simulink model "BESS1_pu"  (R2020b)
settings: Solver=ode1  StartTime=0.0  StopTime=160  FixedStep=Ts  RelTol=1e-3
PostLoadFcn:
  | clc; clear all; close all;
  | 
  | % Modulo 10 - Controle Grid-Forming %
  | 
  | vs_ref = 400;
  | Vnom_rms = vs_ref;
  | Vnom_peak = sqrt(2/3)*Vnom_rms;
  | Pnom =29.75e3;
  | Sbase = Pnom;
  | Vdc = 1400;
  | wnom = 2*pi*60;
  | ron = 0.00088;
  | Ron = ron;
  | %%%% To pu %%%%
  | Vbase = Vnom_rms*sqrt(2);
  | V_LG = Vnom_rms/sqrt(3);
  | Ibase = (Pnom*sqrt(2))/(V_LG*3);
  | 
  | Irms = Pnom/(sqrt(3)*Vnom_rms);                     % Ig rms
  | Inom_peak = Irms*sqrt(2);                           % Ig pico
  | Zbase = Vnom_peak/Inom_peak;                        % Impedancia Base
  | Kconv = Zbase;                                      % Ganho conversor
  | 
  | %%%% LCL Filter Project %%%%
  | fsw = 105*60;%105*60;                                         % switching frequency
  | ripple = 0.05;                                       % current ripple
  | L1 = Vdc/(6*ripple*Inom_peak*fsw);                  % inductor L1
  | R1 = 0.005;                                        % L1 resistance
  | Cbase = 1/(wnom*Kconv);                             % base capacitance
  | Cf = 0.05*Cbase;                                    % filter capacitor
  | Cf = 400e-6;
  | 
  | 
  | % Capacitor DC
  | C_cc_proj = (Sbase/(2*pi*60*Vdc*Vdc*0.05));
  | 
  | % Controladores
  | tau_i = 0.0005;
  | kp_corrente = L1/tau_i
  | ki_corrente = (R1+ron)/tau_i
  | kp_current_pu = kp_corrente/Kconv;                  % Adaptando para pu
  | ki_current_pu = ki_corrente/Kconv;
  | decouple_pu = (wnom*L1+(R1+Ron))/Kconv;
  | 
  | %decouple_i = wnom*L1
  | decouple_v = wnom*Cf
  | decouple_v_pu = (wnom*Cf)*Kconv;
  | 
  | % Controlador CA
  | S_Load = sqrt((25e3)^2+(20e3)^2);
  | Ibase_Load = ((S_Load*sqrt(2))/(V_LG*3))
  | 
  | 
  | a1=2
  | kp_tensao = Cf/(a1*tau_i)
  | Tn = 4*tau_i;
  | ki_tensao = kp_tensao/Tn
  | 
  | % To pu
  | Ica_pu = Pnom/Vdc;
  | %Kcc = Vdc/Iext;
  | 
  | 
  | 
  | 
  | a2=(1+(2/sqrt(2)))
  | kp_tensao2 = Cf/(a2*tau_i)
  | ki_tensao2 = kp_tensao2/Tn
  | 
  | 
  | Ts =25e-6; Ts_Control=Ts;
  | 
  | % PR_ideal_tensao = tf([2*ki_tensao],[1 0 (w^2)]);
  | % PR_ideal_corrente = tf([2*ki_corrente],[1 0 (w^2)]);
  | % figure(1)
  | % bode(PR_ideal_tensao)
  | %
  | % wc = 5;
  | %
  | % PR_real = tf([2*ki_tensao*wc],[1 2*wc (w^2)]);
  | % figure(2)
  | % bode(PR_real)
  | %
  | % wc1 = 1;
  | %
  | % PR_real1 = tf([2*ki_tensao*wc1],[1 2*wc1 (w^2)]);
  | % figure(3)
  | % bode(PR_real1)
InitFcn:
  | clc; clear all; close all;
  | 
  | % Modulo 10 - Controle Grid-Forming %
  | 
  | vs_ref = 400;
  | Vnom_rms = vs_ref;
  | Vnom_peak = sqrt(2/3)*Vnom_rms;
  | Pnom =29.75e3;
  | Sbase = Pnom;
  | Vdc = 1400;
  | wnom = 2*pi*60;
  | ron = 0.00088;
  | Ron = ron;
  | %%%% To pu %%%%
  | Vbase = Vnom_rms*sqrt(2);
  | V_LG = Vnom_rms/sqrt(3);
  | Ibase = (Pnom*sqrt(2))/(V_LG*3);
  | 
  | Irms = Pnom/(sqrt(3)*Vnom_rms);                     % Ig rms
  | Inom_peak = Irms*sqrt(2);                           % Ig pico
  | Zbase = Vnom_peak/Inom_peak;                        % Impedancia Base
  | Kconv = Zbase;                                      % Ganho conversor
  | 
  | %%%% LCL Filter Project %%%%
  | fsw = 105*60;%105*60;                                         % switching frequency
  | ripple = 0.05;                                       % current ripple
  | L1 = Vdc/(6*ripple*Inom_peak*fsw);                  % inductor L1
  | R1 = 0.005;                                        % L1 resistance
  | Cbase = 1/(wnom*Kconv);                             % base capacitance
  | Cf = 0.05*Cbase;                                    % filter capacitor
  | Cf = 400e-6;
  | 
  | 
  | % Capacitor DC
  | C_cc_proj = (Sbase/(2*pi*60*Vdc*Vdc*0.05));
  | 
  | % Controladores
  | tau_i = 0.0005;
  | kp_corrente = L1/tau_i
  | ki_corrente = (R1+ron)/tau_i
  | kp_current_pu = kp_corrente/Kconv;                  % Adaptando para pu
  | ki_current_pu = ki_corrente/Kconv;
  | decouple_pu = (wnom*L1+(R1+Ron))/Kconv;
  | 
  | %decouple_i = wnom*L1
  | decouple_v = wnom*Cf
  | decouple_v_pu = (wnom*Cf)*Kconv;
  | 
  | % Controlador CA
  | S_Load = sqrt((25e3)^2+(20e3)^2);
  | Ibase_Load = ((S_Load*sqrt(2))/(V_LG*3))
  | 
  | 
  | a1=2
  | kp_tensao = Cf/(a1*tau_i)
  | Tn = 4*tau_i;
  | ki_tensao = kp_tensao/Tn
  | 
  | % To pu
  | Ica_pu = Pnom/Vdc;
  | %Kcc = Vdc/Iext;
  | 
  | 
  | 
  | 
  | a2=(1+(2/sqrt(2)))
  | kp_tensao2 = Cf/(a2*tau_i)
  | ki_tensao2 = kp_tensao2/Tn
  | 
  | 
  | Ts =25e-6; Ts_Control=Ts;
  | 
  | % PR_ideal_tensao = tf([2*ki_tensao],[1 0 (w^2)]);
  | % PR_ideal_corrente = tf([2*ki_corrente],[1 0 (w^2)]);
  | % figure(1)
  | % bode(PR_ideal_tensao)
  | %
  | % wc = 5;
  | %
  | % PR_real = tf([2*ki_tensao*wc],[1 2*wc (w^2)]);
  | % figure(2)
  | % bode(PR_real)
  | %
  | % wc1 = 1;
  | %
  | % PR_real1 = tf([2*ki_tensao*wc1],[1 2*wc1 (w^2)]);
  | % figure(3)
  | % bode(PR_real1)
StartFcn:
  | clc; clear all; close all;
  | 
  | % Modulo 10 - Controle Grid-Forming %
  | 
  | vs_ref = 400;
  | Vnom_rms = vs_ref;
  | Vnom_peak = sqrt(2/3)*Vnom_rms;
  | Pnom =29.75e3;
  | Sbase = Pnom;
  | Vdc = 1400;
  | wnom = 2*pi*60;
  | ron = 0.00088;
  | Ron = ron;
  | %%%% To pu %%%%
  | Vbase = Vnom_rms*sqrt(2);
  | V_LG = Vnom_rms/sqrt(3);
  | Ibase = (Pnom*sqrt(2))/(V_LG*3);
  | 
  | Irms = Pnom/(sqrt(3)*Vnom_rms);                     % Ig rms
  | Inom_peak = Irms*sqrt(2);                           % Ig pico
  | Zbase = Vnom_peak/Inom_peak;                        % Impedancia Base
  | Kconv = Zbase;                                      % Ganho conversor
  | 
  | %%%% LCL Filter Project %%%%
  | fsw = 105*60;%105*60;                                         % switching frequency
  | ripple = 0.05;                                       % current ripple
  | L1 = Vdc/(6*ripple*Inom_peak*fsw);                  % inductor L1
  | R1 = 0.005;                                        % L1 resistance
  | Cbase = 1/(wnom*Kconv);                             % base capacitance
  | Cf = 0.05*Cbase;                                    % filter capacitor
  | Cf = 400e-6;
  | 
  | 
  | % Capacitor DC
  | C_cc_proj = (Sbase/(2*pi*60*Vdc*Vdc*0.05));
  | 
  | % Controladores
  | tau_i = 0.0005;
  | kp_corrente = L1/tau_i
  | ki_corrente = (R1+ron)/tau_i
  | kp_current_pu = kp_corrente/Kconv;                  % Adaptando para pu
  | ki_current_pu = ki_corrente/Kconv;
  | decouple_pu = (wnom*L1+(R1+Ron))/Kconv;
  | 
  | %decouple_i = wnom*L1
  | decouple_v = wnom*Cf
  | decouple_v_pu = (wnom*Cf)*Kconv;
  | 
  | % Controlador CA
  | S_Load = sqrt((25e3)^2+(20e3)^2);
  | Ibase_Load = ((S_Load*sqrt(2))/(V_LG*3))
  | 
  | 
  | a1=2
  | kp_tensao = Cf/(a1*tau_i)
  | Tn = 4*tau_i;
  | ki_tensao = kp_tensao/Tn
  | 
  | % To pu
  | Ica_pu = Pnom/Vdc;
  | %Kcc = Vdc/Iext;
  | 
  | 
  | 
  | 
  | a2=(1+(2/sqrt(2)))
  | kp_tensao2 = Cf/(a2*tau_i)
  | ki_tensao2 = kp_tensao2/Tn
  | 
  | 
  | Ts =25e-6; Ts_Control=Ts;
  | 
  | % PR_ideal_tensao = tf([2*ki_tensao],[1 0 (w^2)]);
  | % PR_ideal_corrente = tf([2*ki_corrente],[1 0 (w^2)]);
  | % figure(1)
  | % bode(PR_ideal_tensao)
  | %
  | % wc = 5;
  | %
  | % PR_real = tf([2*ki_tensao*wc],[1 2*wc (w^2)]);
  | % figure(2)
  | % bode(PR_real)
  | %
  | % wc1 = 1;
  | %
  | % PR_real1 = tf([2*ki_tensao*wc1],[1 2*wc1 (w^2)]);
  | % figure(3)
  | % bode(PR_real1)
undefined symbols (not defined in the file): DiscIntNeverNeededParam, I, Ion, Left, Lithium, ph, type, V
libraries: powerlib x18, powerlib_meascontrol x16, rtlab x6, artemis x2, eePowerMeasurement x2, rteventslib x2, ssn_inverter_model x1, electricdrivelib x1
(part 1 of 2)
settings Model: ARTEMISmethode_block_infos=$$__separator__$$BESS1_pu/ARTEMIS Guide$$__separator__$$  Creator=Lafae  LastModifiedBy=lafae
settings DataIOCC: SaveOutput=off  SaveTime=off  ReturnWorkspaceOutputs=off
settings OptimizationCC: BlockReduction=off  OptimizeBlockIOStorage=off  BufferReuse=off  GlobalBufferReuse=off  ExpressionFolding=off  LocalBlockOutputs=off  OptimizeDataStoreBuffers=off  BusAssignmentInplaceUpdate=off
settings DebuggingCC: ArithmeticOperatorsInVariantConditions=warning
settings SFSimCC: CustomCodeUndefinedFunction=UseInterfaceOnly

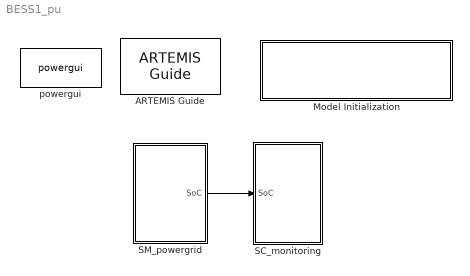
== system BESS1_pu ==
  ARTEMIS Guide : artemis/ARTEMIS/ARTEMIS Guide  Tag=art7.5  Description=New ARTEMiS block v 7.5b (R2015b+)  lock=on  Ts=Ts  ssn=on  opt=art5  dyna=off  nb_perm=4  RT_fullcomp=off  ssn_itvc=off  ssn_ivic=off  ssn_ext=off  ssn_solver=Art5  iter_type=iSWITCH and iMOV only (default)  ssn_ImpulseLoopBlockedStateUpdate=5  ssn_mov_iter_number=5  ssn_switch_iter_number=3  ssn_lu_or_ldlt=LU (more robust)  ssn_nib_type_verify=on  ssn_use_lu=on  ssn_use_ldlt=off  ssn_impulse=on  ssn_quasimpulse=off  ssn_impulse_loop=5  paraExtinctionThy=off  Thy_Impulse=on  dtc=Off  dtc_opt=normal  ao=off  simtype=off  ct_mac=off  lin_mov=off  lsp=[0.001 2]  spike_skip=Disabled  dtc_extra=1  dtc_sws=normal  dtc_pied=0.5  SPSRulesBlock=SPSRules  tre=off  ctmm=off  LF=off  dpl_type=ARTEMiS DPL  rlc_type=off  custom_type=off  para=on  ssn_full_iteration=off  ssn_init_cond=block only
  Model Initialization : Subsystem  AncestorBlock=artemis/Tools /Misc/Model Initialization  mask(Model Functions){InitFcnX=|, prel=off, posl=on, inif=on, strf=on}
      mask InitFcnX=|
      | clc; clear all; close all;
      |
      | % Modulo 10 - Controle Grid-Forming %
      |
      | vs_ref = 400;
      | Vnom_rms = vs_ref;
      | Vnom_peak = sqrt(2/3)*Vnom_rms;
      | Pnom =29.75e3;
      | Sbase = Pnom;
      | Vdc = 1400;
      | wnom = 2*pi*60;
      | ron = 0.00088;
      | Ron = ron;
      | %%%% To pu %%%%
      | Vbase = Vnom_rms*sqrt(2);
      | V_LG = Vnom_rms/sqrt(3);
      | Ibase = (Pnom*sqrt(2))/(V_LG*3);
      |
      | Irms = Pnom/(sqrt(3)*Vnom_rms);                     % Ig rms
      | Inom_peak = Irms*sqrt(2);                           % Ig pico
      | Zbase = Vnom_peak/Inom_peak;                        % Impedancia Base
      | Kconv = Zbase;                                      % Ganho conversor
      |
      | %%%% LCL Filter Project %%%%
      | fsw = 105*60;%105*60;                                         % switching frequency
      | ripple = 0.05;                                       % current ripple
      | L1 = Vdc/(6*ripple*Inom_peak*fsw);                  % inductor L1
      | R1 = 0.005;                                        % L1 resistance
      | Cbase = 1/(wnom*Kconv);                             % base capacitance
      | Cf = 0.05*Cbase;                                    % filter capacitor
      | Cf = 400e-6;
      |
      |
      | % Capacitor DC
      | C_cc_proj = (Sbase/(2*pi*60*Vdc*Vdc*0.05));
      |
      | % Controladores
      | tau_i = 0.0005;
      | kp_corrente = L1/tau_i
      | ki_corrente = (R1+ron)/tau_i
      | kp_current_pu = kp_corrente/Kconv;                  % Adaptando para pu
      | ki_current_pu = ki_corrente/Kconv;
      | decouple_pu = (wnom*L1+(R1+Ron))/Kconv;
      |
      | %decouple_i = wnom*L1
      | decouple_v = wnom*Cf
      | decouple_v_pu = (wnom*Cf)*Kconv;
      |
      | % Controlador CA
      | S_Load = sqrt((25e3)^2+(20e3)^2);
      | Ibase_Load = ((S_Load*sqrt(2))/(V_LG*3))
      |
      |
      | a1=2
      | kp_tensao = Cf/(a1*tau_i)
      | Tn = 4*tau_i;
      | ki_tensao = kp_tensao/Tn
      |
      | % To pu
      | Ica_pu = Pnom/Vdc;
      | %Kcc = Vdc/Iext;
      |
      |
      |
      |
      | a2=(1+(2/sqrt(2)))
      | kp_tensao2 = Cf/(a2*tau_i)
      | ki_tensao2 = kp_tensao2/Tn
      |
      |
      | Ts =25e-6; Ts_Control=Ts;
      |
      | % PR_ideal_tensao = tf([2*ki_tensao],[1 0 (w^2)]);
      | % PR_ideal_corrente = tf([2*ki_corrente],[1 0 (w^2)]);
      | % figure(1)
      | % bode(PR_ideal_tensao)
      | %
      | % wc = 5;
      | %
      | % PR_real = tf([2*ki_tensao*wc],[1 2*wc (w^2)]);
      | % figure(2)
      | % bode(PR_real)
      | %
      | % wc1 = 1;
      | %
      | % PR_real1 = tf([2*ki_tensao*wc1],[1 2*wc1 (w^2)]);
      | % figure(3)
      | % bode(PR_real1)
      mask prompts: InitFcnX "Initialisation"; prel "Preload Function"; posl "PostLoad Function"; inif "InitFcn"; strf "StartFcn"
      mask init:
      | currentBlock = gcb;
      | root = bdroot(currentBlock);
      | 
      | if ~strcmp(get_param(root,'BlockDiagramType'),'library')
      |     if prel==1
      |         set_param(root, 'PreLoadFcn', InitFcnX);
      |     else
      |         set_param(root, 'PreLoadFcn', '');
      |     end
      |     if inif==1
      |         set_param(root, 'InitFcn', InitFcnX);
      |     else
      |         set_param(root, 'InitFcn', '');
      |     end
      |     if strf==1
      |         set_param(root, 'StartFcn', InitFcnX);
      |     else
      |         set_param(root, 'StartFcn', '');
      |     end
      |     if posl==1
      |         set_param(root, 'PostLoadFcn', InitFcnX);
      |     else
      |         set_param(root, 'PostLoadFcn', '');
      |     end
      | end
      | 
      | pos = get_param(currentBlock, 'Position');
      | width = pos(3) - pos(1); height = pos(4) - pos(2);
      | txt = [ upper(root) '\n' '- InitFcn. . . . . '  get_param(root, 'InitFcn') ];
      settings: CopyFcn=set_param(gcb,'LinkStatus','inactive')
      mask Display: text(5, height*0.5, txt, 'horizontalAlignment', 'left', 'verticalAlignment', 'middle') ;
  SC_monitoring : Subsystem
  SM_powergrid : Subsystem
  powergui : powerlib/powergui  Priority=1  SimulationMode=Discrete  SampleTime=Ts  frequency=60  Iterations=50  frequencyindice=0  Pbase=100e6  ErrMax=1e-4  UnitsV=kV  UnitsW=MW  buscounter=0  FunctionMessages=off  echomessages=off  EnableUseOfTLC=off  CurrentSourceSwitches=off  DisableSnubberDevices=off  DisableRonSwitches=off  DisableVfSwitches=off  DisplayEquations=off  AutomaticDiscreteSolvers=off  SolverType=Tustin/Backward Euler (TBE)  Interpol=off  ExternalGateDelay=off  methode=off  Ts=100  x0status=blocks  SPID=off  SwTol=0  HookPort=off  NonlinearTolerance=1e-4  nMaxIteration=100  ContinueOnMaxIteration=off  RestoreLinks=warning  ResistiveCurrentMeasurement=off  Frange=[0:2:500]  Ylog=off  Xlog=on  ShowGrid=off  save=off  variable=ZData  structure=0  ZoomFFT=off  StartTime=0.0  cycles=1  DisplayStyle=1  fundamental=60  FreqAxis=off  MaxFrequency=1000  frequencyindicesteady=1  RmsSteady=1  display=off
  wires:
  SM_powergrid/1(SoC) -> SC_monitoring/1(SoC)

== system BESS1_pu/Model Initialization ==

== system BESS1_pu/SC_monitoring ==
  SoC : Inport
  OpComm : rtlab/OpComm  nbport=1  groupe_acq=1  subsys_rate=0  st=0  Synchronization=on  Interpolation=on  Threshold=1.0  Missed_Data=off  Sim_Time=off  Samples=off  dynSigOut=off  from_console=0  warning_done=off  writeOpCommFile=off  Offset=off
      settings: SourceProductName=RT-LAB
  SoC_m : Scope
  wires:
  SoC/1 -> OpComm/1
  OpComm/1 -> SoC_m/1

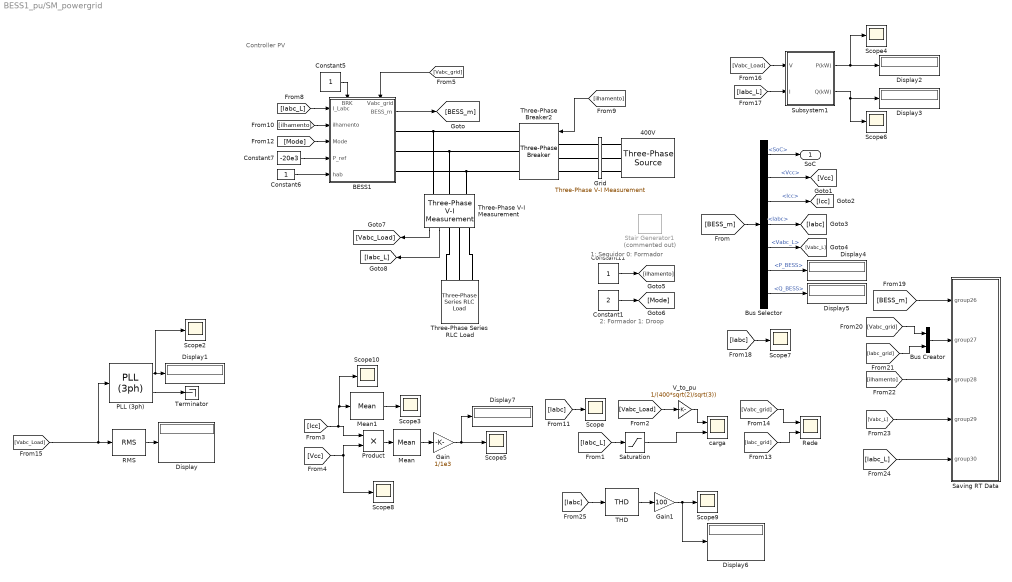
== system BESS1_pu/SM_powergrid ==
  note: Controller PV
  note: 1: Seguidor
      | 0: Formador
  note: 2: Formador
      | 1: Droop
  "400V " : powerlib/Electrical Sources/Three-Phase Source  InternalConnection=Yg  VoltagePhases=off  Voltage=400  PhaseAngle=0  Voltage_phases=[25e3 25e3 25e3]/sqrt(3)  PhaseAngles_phases=[0 -120 +120]  Frequency=60  NonIdealSource=on  SpecifyImpedance=on  Resistance=0.8929  Inductance=16.58e-3  ShortCircuitLevel=2500e6  BaseVoltage=400  XRratio=7  BusType=swing  Pref=0  Qref=0  Prefabc=[10e3, 10e3, 10e3]  Qrefabc=[0, 0, 0]  Qmin=-inf  Qmax=inf
  BESS1 : Subsystem  mask{Parameter1=0, Vdc=1400}
      mask prompts: Parameter1 "Active Power"; Vdc "Voltage BESS"
      settings: PortSchema="{\"entries\":[{\"content\":{\"sides\":[{\"content\":{\"connectorIds\":[\"In1\",\"In2\",\"In3\",\"In4\",\"In5\"]},\"type\":\"ConnectorPlacement.EquallySpacedRectSide\",\"uuid\":\"b852895c-1a88-46a2-b5c3-3793c2bbfa50\"},{\"content\":{\"connectorIds\":[\"Out1\",\"RConn1\",\"RConn2\",\"RConn3\"],\"side\":\"RIGHT\"},\"type\":\"ConnectorPlacement.EquallySpacedRectSide\",\"uuid\":\"623e2f3e-e54c-4c45-bbde-85363be8e45a\"},{\"content\":{\"connectorIds\":[\"In6\",\"In7\"],\"side\":\"TOP\"},\"type\":\"ConnectorPlacement.EquallySpacedRectSide\",\"uuid\":\"4361bef1-4271-4d53-bf17-8738c4288524\"},{\"content\":{\"connectorIds\":[],\"side\":\"BOTTOM\"},\"type\":\"ConnectorPlacement.EquallySpacedRectSide\",\"uuid\":\"fccd725a-212e-4f4d-86e2-af3e4cb1e181\"},{\"content\":{\"connectorIds\":[],\"side\":\"HIDDEN\"},\"type\":\"ConnectorPlacement.EquallySpacedRectSide\",\"uuid\":\"18fd8fa2-4388-4fef-bc52-b43f49f76590\"}]},\"type\":\"ConnectorPlacement.EquallySpacedConnector\",\"uuid\":\"f9b6b572-f2f1-4797-9202-fef1628d084a\"}],\"packageUris\":[\"http://schema.mathworks.com/mf0/Connector/R2020b\"],\"version\":\"1.0\"}"
      mask Display:
      | %image('$imagefile'); % Use "Edit Image" on toolstrip to change.
      | 
      | port_label('input',1,'I_Labc')
      | port_label('input',2,'ilha')
      | port_label('input',3,'Mode')
      | port_label('input',4,'P_ref')
      | port_label('input',5,'hab')
      | port_label('input',6,'BRK')
      | 
      | %output
      | port_label('output',1,'PBESS_m')
      | 
      | %electrical
      | port_label('Rconn',1,'Va')
      | port_label('Rconn',2,'Vb')
      | port_label('Rconn',3,'Vc')
  Bus Creator : BusCreator  Inputs=2
  Bus Selector : BusSelector  OutputSignals=SoC,Vcc,Icc,Iabc,Vabc_L,P_BESS,Q_BESS
  Constant1 : Constant  Value=2
  Constant11 : Constant
  Constant5 : Constant
  Constant6 : Constant
  Constant7 : Constant  Value=-20e3
  Display{,1..7} (8 alike) : Display
  Gain : Gain  Gain=1/1e3
  Gain1 : Gain  Gain=100
  Grid : powerlib/Measurements/Three-Phase V-I Measurement  VoltageMeasurement=phase-to-ground  SetLabelV=on  LabelV=Vabc_grid  Vpu=off  VpuLL=off  CurrentMeasurement=yes  SetLabelI=on  LabelI=Iabc_grid  Ipu=off  Pbase=100e6  Vbase=500e3  OutputType=Complex  PhasorSimulation=off  PSBequivalent=0
  Mean : powerlib_meascontrol/Measurements/Mean  Freq=60  Vinit=0  Ts=0
  Mean1 : powerlib_meascontrol/Measurements/Mean  Freq=60  Vinit=0  Ts=0
  PLL (3ph) : powerlib_meascontrol/PLL/PLL (3ph)  Fmin=45  Par_Init="[-0.57  60]"  ParK=[180, 3200, 1]  TcD=Ts  MaxRateChangeFreq=12  FilterCutOffFreq=25  Ts=Ts  AGC=on
  Product : Product
  RMS : powerlib_meascontrol/Measurements/RMS  TrueRMS=on  Freq=60  RMSInit=1  Ts=Ts
  Rede : Scope  NumInputPorts=2
  Saturation : Saturate  UpperLimit=100  LowerLimit=-100
  Saving RT Data : Subsystem  mask{Ts=Ts, Decimation26=3, varname26=BESS_m, Filename26=BESS.mat, nls26=38, ld26=40, Decimation27=3, varname27=Grid_m, Filename27=Grid.mat, nls27=15, ld27=40, Decimation28=3, varname28=cmd_isla, Filename28=cmd_BRK.mat, nls28=19, ld28=40, Decimation29=3, varname29=Vabc_L, Filename29=Vabc_L.mat, nls29=19, ld29=40, Decimation30=3, varname30=Iabc_L, Filename30=Iabc_L.mat, nls30=20, ld30=40}
      mask prompts: Ts "Ts (s)"; Decimation26 "Decimation factor"; varname26 "Variable name"; Filename26 "FileName"; nls26 "Number of logged signals"; ld26 "Logging duration (s)"; Decimation27 "Decimation factor"; varname27 "Variable name"; Filename27 "FileName"; nls27 "Number of logged signals"; ld27 "Logging duration (s)"; Decimation28 "Decimation factor"; varname28 "Variable name"; Filename28 "FileName"; nls28 "Number of logged signals"; ld28 "Logging duration (s)"; Decimation29 "Decimation factor"; varname29 "Variable name"; Filename29 "FileName"; nls29 "Number of logged signals"; ld29 "Logging duration (s)"; Decimation30 "Decimation factor"; varname30 "Variable name"; Filename30 "FileName"; nls30 "Number of logged signals"; ld30 "Logging duration (s)"
      mask help: This block contains the 5 groups of OpWriteFile (26, 27, 28 29 and 30) blocks that write signals to a binary file (.mat), files that are in the binary data container format that MATLAB uses.
      mask TypeOptions Decimation26: OpWriteFile26/Decimation
      mask TypeOptions varname26: OpWriteFile26/varname
      mask TypeOptions Filename26: OpWriteFile26/Filename
      mask TypeOptions Decimation27: OpWriteFile27/Decimation
      mask TypeOptions varname27: OpWriteFile27/varname
      mask TypeOptions Filename27: OpWriteFile27/Filename
      mask TypeOptions Decimation28: OpWriteFile28/Decimation
      mask TypeOptions varname28: OpWriteFile28/varname
      mask TypeOptions Filename28: OpWriteFile28/Filename
      mask TypeOptions Decimation29: OpWriteFile29/Decimation
      mask TypeOptions varname29: OpWriteFile29/varname
      mask TypeOptions Filename29: OpWriteFile29/Filename
      mask TypeOptions Decimation30: OpWriteFile30/Decimation
      mask TypeOptions varname30: OpWriteFile30/varname
      mask TypeOptions Filename30: OpWriteFile30/Filename
      mask DialogControl DescGroupVar Prompt: Saving RT Data
      mask DialogControl Container4 Prompt: Group 26
      mask DialogControl Container9 Prompt: Group 27
      mask DialogControl Container10 Prompt: Group 28
      mask DialogControl Container11 Prompt: Group 29
      mask DialogControl Container12 Prompt: Group 30
  Scope{,2..10} (10 alike) : Scope
  Stair Generator1 : powerlib_meascontrol/Pulse & Signal Generators/Stair Generator  Commented=on  t=[0, 5, 30, 66]  e=[0, 1, 0, 1]  Ts=0
  Subsystem1 : Subsystem
  THD : powerlib_meascontrol/Measurements/THD  Freq=60  Ts=0
  Terminator : Terminator
  Three-Phase Series RLC Load : powerlib/Elements/Three-Phase Series RLC Load  LConnTagsString=A|B|C  Configuration=Y (grounded)  NominalVoltage=400  Vabc=[1e3 1e3 1e3]  Vabcp=[1e3 1e3 1e3]  NominalFrequency=60  UnbalancedPower=off  ActivePower=25e3  InductivePower=20e3  CapacitivePower=0  Pabc=[10e3 9e3 11e3]  QLabc=[100 90 110]  QCabc=[100 90 110]  Pabcp=[10e3 9e3 11e3]  QLabcp=[100 90 110]  QCabcp=[100 90 110]  Measurements=None  LoadType=constant Z
  Three-Phase V-I Measurement : powerlib/Measurements/Three-Phase V-I Measurement  VoltageMeasurement=phase-to-ground  SetLabelV=off  LabelV=Vabc  Vpu=off  VpuLL=off  CurrentMeasurement=yes  SetLabelI=off  LabelI=Iabc  Ipu=off  Pbase=100e6  Vbase=500e3  OutputType=Complex  PhasorSimulation=off  PSBequivalent=0
  Three-Phase Breaker2 : powerlib/Elements/Three-Phase Breaker  InitialState=open  SwitchA=on  SwitchB=on  SwitchC=on  SwitchTimes=[10]  External=on  BreakerResistance=0.001  SnubberResistance=1e6  SnubberCapacitance=inf  Measurements=None
  V_to_pu : Gain  Gain=1/(400*sqrt(2)/sqrt(3))  SaturateOnIntegerOverflow=on  OutDataTypeStr=Inherit: Same as input  ParamDataTypeStr=Inherit: Same as input
  carga : Scope  NumInputPorts=2
  SoC : Outport
  wires:
  [Icc] -> Scope10/1, Mean1/1, Product/1
  [Vcc] -> Scope8/1, Product/2
  Product/1 -> Mean/1
  Mean/1 -> Gain/1
  Gain/1 -> Display7/1, Scope5/1
  [ilhamento] -> Three-Phase Breaker2/1
  [Iabc] -> Scope/1
  [Iabc_grid] -> Rede/2
  [Vabc_grid] -> Rede/1
  Constant11/1 -> [ilhamento]
  BESS1/1(BESS_m) -> [BESS_m]
  [BESS_m] -> Bus Selector/1
  Bus Selector/1 -> SoC/1  "<SoC>"
  Bus Selector/2 -> [Vcc]  "<Vcc>"
  Bus Selector/3 -> [Icc]  "<Icc>"
  Bus Selector/4 -> [Iabc]  "<Iabc>"
  Bus Selector/5 -> [Vabc_L]  "<Vabc_L>"
  Constant1/1 -> [Mode]
  Constant5/1 -> BESS1/6(BRK)
  [Iabc_L] -> BESS1/1(I_Labc)
  [ilhamento] -> BESS1/2(ilhamento)
  [Mode] -> BESS1/3(Mode)
  Constant7/1 -> BESS1/4(P_ref)
  Constant6/1 -> BESS1/5(hab)
  [Vabc_Load] -> PLL (3ph)/1, RMS/1
  RMS/1 -> Display/1
  PLL (3ph)/2 -> Terminator/1
  PLL (3ph)/1 -> Scope2/1, Display1/1
  Three-Phase V-I Measurement/1 -> [Vabc_Load]
  Three-Phase V-I Measurement/2 -> [Iabc_L]
  [Iabc_L] -> Saturation/1
  Saturation/1 -> carga/2
  [Vabc_Load] -> Subsystem1/1(V)
  [Iabc_L] -> Subsystem1/2(I)
  Subsystem1/1(P(kW)) -> Scope4/1, Display2/1
  Subsystem1/2(Q(kW)) -> Display3/1, Scope6/1
  [Iabc] -> Scope7/1
  Bus Selector/6 -> Display4/1  "<P_BESS>"
  Bus Selector/7 -> Display5/1  "<Q_BESS>"
  Mean1/1 -> Scope3/1
  [BESS_m] -> Saving RT Data/1(group26)
  [Iabc_grid] -> Bus Creator/2
  [Vabc_grid] -> Bus Creator/1
  Bus Creator/1 -> Saving RT Data/2(group27)
  [ilhamento] -> Saving RT Data/3(group28)
  [Vabc_L] -> Saving RT Data/4(group29)
  [Iabc_L] -> Saving RT Data/5(group30)
  [Iabc] -> THD/1
  THD/1 -> Gain1/1
  Gain1/1 -> Display6/1, Scope9/1
  [Vabc_grid] -> BESS1/7(Vabc_grid)
  [Vabc_Load] -> V_to_pu/1
  V_to_pu/1 -> carga/1
  connections:
  Three-Phase V-I Measurement/LConn2 -- Three-Phase Breaker2/RConn2 -- BESS1/RConn2
  Three-Phase V-I Measurement/LConn1 -- BESS1/RConn1 -- Three-Phase Breaker2/RConn1
  Grid/LConn2 -- Three-Phase Breaker2/LConn2
  Grid/LConn1 -- Three-Phase Breaker2/LConn1
  Three-Phase Breaker2/LConn3 -- Grid/LConn3
  "400V "/RConn2 -- Grid/RConn2
  "400V "/RConn3 -- Grid/RConn3
  "400V "/RConn1 -- Grid/RConn1
  Three-Phase V-I Measurement/LConn3 -- BESS1/RConn3 -- Three-Phase Breaker2/RConn3
  Three-Phase Series RLC Load/LConn1 -- Three-Phase V-I Measurement/RConn1
  Three-Phase Series RLC Load/LConn2 -- Three-Phase V-I Measurement/RConn2
  Three-Phase Series RLC Load/LConn3 -- Three-Phase V-I Measurement/RConn3

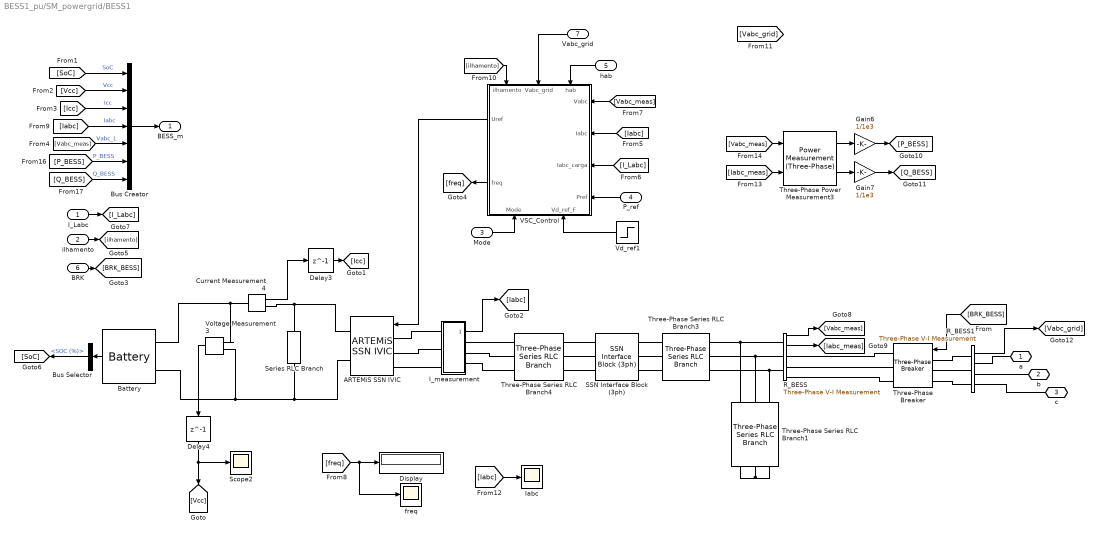
== system BESS1_pu/SM_powergrid/BESS1 ==
  I_Labc : Inport
  ilhamento : Inport  Port=2
  Mode : Inport  Port=3
  P_ref : Inport  Port=4
  hab : Inport  Port=5
  BRK : Inport  Port=6
  Vabc_grid : Inport  Port=7
  ARTEMiS SSN IVIC : ssn_inverter_model/ARTEMiS SSN IVIC  Arms=3  SnubberResistance=800  SnubberCapacitance=inf  Device=IGBT / Diodes  Ron=0.00088  Lon=0  ForwardVoltages=[0.001 0.001]  ForwardVoltage=0  GTOparameters=[ 10e-6 , 20e-6 ]  IGBTparameters=[ 1e-6 , 2e-6 ]*0  Measurements=None  Measurements_2=None  converterType=Rectifier
  Battery : electricdrivelib/Extra Sources/Battery  BatType=Lithium-Ion  ShowTempParam=off  ThermalPreset=no  ShowAgeParam=off  NomV=1400  NomQ=2  SOC=50  Batt_Tr=30  PresetModel=on  MaxQ=2  MinV=1050  FullV=1629.582  Dis_rate=0.86957  R=7  Normal_OP=1.8087  expZone="[1512.5402     0.09826087]"  current=[8 23 32.5]  Units=Time  Tci=20  NomT=20  T2=-30  MaxQ2=4.8  FullV2=7.1  Normal_OP2=5.655  expZone2="[6.58           1]"  Rca=0.6  ti=2000  Dp=0  Neq0=0  Tsim=1e6  Ta1=25  Qeol=5.4*0.9  Reol=0.013333*1.2  Char_age=[2.3478, 3]  Dis_age=[2.3478, 10]  N1=1500  N2=10500  N3=1000  N4=1400  Ta2=45  N5=950
  Bus Creator : BusCreator  Inputs=7
  Bus Selector : BusSelector  OutputSignals=SOC (%)
  Current Measurement4 : powerlib/Measurements/Current Measurement  PhasorSimulation=off  OutputType=Complex  PSBequivalent=0
  Delay3 : Delay  DelayLength=1  InitialCondition=0
  Delay4 : Delay  DelayLength=1  InitialCondition=0
  Display : Display
  Gain6 : Gain  Gain=1/1e3
  Gain7 : Gain  Gain=1/1e3
  I_measurement : Subsystem
  Iabc : Scope
  R_BESS : powerlib/Measurements/Three-Phase V-I Measurement  VoltageMeasurement=phase-to-ground  SetLabelV=off  LabelV=Vabc_meas  Vpu=off  VpuLL=off  CurrentMeasurement=yes  SetLabelI=off  LabelI=Iabc_meas  Ipu=off  Pbase=100e6  Vbase=400*sqrt(3/2)  OutputType=Complex  PhasorSimulation=off  PSBequivalent=0
  R_BESS1 : powerlib/Measurements/Three-Phase V-I Measurement  VoltageMeasurement=phase-to-ground  SetLabelV=off  LabelV=Vabc_meas  Vpu=off  VpuLL=off  CurrentMeasurement=no  SetLabelI=off  LabelI=Iabc_meas  Ipu=off  Pbase=100e6  Vbase=400*sqrt(3/2)  OutputType=Complex  PhasorSimulation=off  PSBequivalent=0
  SSN Interface Block (3ph) : artemis/SSN/Nodal Interface Blocks/SSN Interface Block (3ph)  nb_phase=3  nb_port=2  p1_type=I-type(Left)  p2_type=V-type (Right)  p3_type=V-type(Left)  p4_type=V-type(Left)  p5_type=V-type(Left)  p6_type=V-type(Left)  p7_type=V-type(Left)  p8_type=V-type(Left)  p9_type=V-type(Left)  p10_type=V-type(Left)  p11_type=V-type(Left)  p12_type=V-type(Left)  p13_type=V-type(Left)  p14_type=V-type(Left)  p15_type=V-type(Left)  p16_type=V-type(Left)  I_port_shunt_resistance=1e9
  Scope2 : Scope
  Series RLC Branch : powerlib/Elements/Series RLC Branch  LConnTagsString=__new0  RConnTagsString=__new0  BranchType=C  Resistance=0.001  Inductance=1e-3  SetiL0=off  InitialCurrent=0  Capacitance=C_cc_proj  Setx0=off  InitialVoltage=0  Measurements=None
  Three-Phase Series RLC Branch1 : powerlib/Elements/Three-Phase Series RLC Branch  LConnTagsString=A|B|C  RConnTagsString=A|B|C  BranchType=C  Resistance=0.019  Inductance=0.0001  Capacitance=Cf  Measurements=None
  Three-Phase Series RLC Branch3 : powerlib/Elements/Three-Phase Series RLC Branch  LConnTagsString=A|B|C  RConnTagsString=A|B|C  BranchType=L  Resistance=0.001  Inductance=L1  Capacitance=1e-6  Measurements=None
  Three-Phase Series RLC Branch4 : powerlib/Elements/Three-Phase Series RLC Branch  LConnTagsString=A|B|C  RConnTagsString=A|B|C  BranchType=R  Resistance=R1  Inductance=1e-3  Capacitance=1e-6  Measurements=None
  Three-Phase Breaker : powerlib/Elements/Three-Phase Breaker  InitialState=open  SwitchA=on  SwitchB=on  SwitchC=on  SwitchTimes=[10]  External=on  BreakerResistance=0.001  SnubberResistance=1e6  SnubberCapacitance=inf  Measurements=None
  Three-Phase Power Measurement3 : eePowerMeasurement/Power Measurement (Three-Phase)  LabelModeActiveChoice=Continuous  F=60  K=[1]  Seq=Positive  Ts=0
      settings: SourceProductBaseCode=PS
  VSC_Control : Subsystem
      settings: PortSchema="{\"entries\":[{\"content\":{\"sides\":[{\"content\":{\"connectorIds\":[\"In1\",\"In2\",\"In3\",\"In4\"]},\"type\":\"ConnectorPlacement.EquallySpacedRectSide\",\"uuid\":\"583d4136-36a7-44c3-b823-b6f793727c7c\"},{\"content\":{\"connectorIds\":[\"Out1\",\"Out2\"],\"side\":\"RIGHT\"},\"type\":\"ConnectorPlacement.EquallySpacedRectSide\",\"uuid\":\"9b5dc4aa-828f-419e-b77b-06d9327907c6\"},{\"content\":{\"connectorIds\":[\"In5\",\"In6\",\"In7\"],\"side\":\"TOP\"},\"type\":\"ConnectorPlacement.EquallySpacedRectSide\",\"uuid\":\"a1a84364-4619-40e4-9faa-434e81a4ea85\"},{\"content\":{\"connectorIds\":[\"In8\",\"In9\"],\"side\":\"BOTTOM\"},\"type\":\"ConnectorPlacement.EquallySpacedRectSide\",\"uuid\":\"dc0d4129-e689-4c31-a594-460b7908aaf8\"},{\"content\":{\"connectorIds\":[],\"side\":\"HIDDEN\"},\"type\":\"ConnectorPlacement.EquallySpacedRectSide\",\"uuid\":\"fa987225-f4ca-42f4-a5dc-7493b019c0f6\"}]},\"type\":\"ConnectorPlacement.EquallySpacedConnector\",\"uuid\":\"39c668ab-a659-4ab9-9d2d-f3653e377efe\"}],\"packageUris\":[\"http://schema.mathworks.com/mf0/Connector/R2020b\"],\"version\":\"1.0\"}"
  Vd_ref1 : Step  Time=0.01  SampleTime=0
  Voltage Measurement3 : powerlib/Measurements/Voltage Measurement  PhasorSimulation=off  OutputType=Complex  PSBequivalent=0
  freq : Scope
  a : PMIOPort  Side=Right
  b : PMIOPort  Port=2  Side=Right
  c : PMIOPort  Port=3  Side=Right
  BESS_m : Outport
  wires:
  R_BESS/2 -> [Iabc_meas]
  R_BESS/1 -> [Vabc_meas]
  P_ref/1 -> VSC_Control/4(Pref)
  hab/1 -> VSC_Control/5(hab)
  Mode/1 -> VSC_Control/9(Mode)
  [Vcc] -> Bus Creator/2  "Vcc"
  [SoC] -> Bus Creator/1  "SoC"
  [Vabc_meas] -> Bus Creator/5  "Vabc_L"
  [Iabc] -> Bus Creator/4  "Iabc"
  [Icc] -> Bus Creator/3  "Icc"
  I_Labc/1 -> [I_Labc]
  Bus Creator/1 -> BESS_m/1
  Bus Selector/1 -> [SoC]  "<SOC (%)>"
  ilhamento/1 -> [ilhamento]
  [I_Labc] -> VSC_Control/3(Iabc_carga)
  Voltage Measurement3/1 -> Delay4/1
  [Vabc_meas] -> VSC_Control/1(Vabc)
  VSC_Control/2(freq) -> [freq]
  Battery/1 -> Bus Selector/1
  [Iabc] -> VSC_Control/2(Iabc)
  [BRK_BESS] -> Three-Phase Breaker/1
  I_measurement/1(Iabc) -> [Iabc]
  BRK/1 -> [BRK_BESS]
  Current Measurement4/1 -> Delay3/1
  Delay3/1 -> [Icc]
  VSC_Control/1(Uref) -> ARTEMiS SSN IVIC/1
  [Iabc] -> Iabc/1
  [ilhamento] -> VSC_Control/7(ilhamento)
  [freq] -> Display/1, freq/1
  Vd_ref1/1 -> VSC_Control/8(Vd_ref_F)
  Delay4/1 -> [Vcc], Scope2/1
  Three-Phase Power Measurement3/1 -> Gain6/1
  Three-Phase Power Measurement3/2 -> Gain7/1
  Gain7/1 -> [Q_BESS]
  Gain6/1 -> [P_BESS]
  [Iabc_meas] -> Three-Phase Power Measurement3/2
  [Vabc_meas] -> Three-Phase Power Measurement3/1
  [P_BESS] -> Bus Creator/6  "P_BESS"
  [Q_BESS] -> Bus Creator/7  "Q_BESS"
  R_BESS1/1 -> [Vabc_grid]
  Vabc_grid/1 -> VSC_Control/6(Vabc_grid)
  connections:
  R_BESS/RConn1 -- Three-Phase Breaker/RConn1
  R_BESS/RConn2 -- Three-Phase Breaker/RConn2
  Current Measurement4/RConn1 -- Series RLC Branch/LConn1 -- ARTEMiS SSN IVIC/RConn1
  SSN Interface Block (3ph)/RConn3 -- Three-Phase Series RLC Branch3/LConn3
  Three-Phase Series RLC Branch4/RConn2 -- SSN Interface Block (3ph)/LConn2
  Three-Phase Series RLC Branch1/LConn1 -- R_BESS/LConn1 -- Three-Phase Series RLC Branch3/RConn1
  I_measurement/LConn3 -- ARTEMiS SSN IVIC/LConn3
  Three-Phase Series RLC Branch4/RConn1 -- SSN Interface Block (3ph)/LConn1
  Three-Phase Series RLC Branch1/RConn2 -- Three-Phase Series RLC Branch1/RConn3 -- Three-Phase Series RLC Branch1/RConn1
  I_measurement/RConn1 -- Three-Phase Series RLC Branch4/LConn1
  Three-Phase Series RLC Branch3/LConn1 -- SSN Interface Block (3ph)/RConn1
  Three-Phase Series RLC Branch1/LConn2 -- R_BESS/LConn2 -- Three-Phase Series RLC Branch3/RConn2
  I_measurement/RConn2 -- Three-Phase Series RLC Branch4/LConn2
  Three-Phase Series RLC Branch4/RConn3 -- SSN Interface Block (3ph)/LConn3
  SSN Interface Block (3ph)/RConn2 -- Three-Phase Series RLC Branch3/LConn2
  I_measurement/RConn3 -- Three-Phase Series RLC Branch4/LConn3
  Three-Phase Series RLC Branch1/LConn3 -- R_BESS/LConn3 -- Three-Phase Series RLC Branch3/RConn3
  Voltage Measurement3/LConn2 -- Battery/LConn2 -- Series RLC Branch/RConn1 -- ARTEMiS SSN IVIC/RConn2
  I_measurement/LConn1 -- ARTEMiS SSN IVIC/LConn1
  I_measurement/LConn2 -- ARTEMiS SSN IVIC/LConn2
  Voltage Measurement3/LConn1 -- Battery/LConn1 -- Current Measurement4/LConn1
  R_BESS/RConn3 -- Three-Phase Breaker/RConn3
  R_BESS1/LConn2 -- Three-Phase Breaker/LConn2
  R_BESS1/LConn1 -- Three-Phase Breaker/LConn1
  R_BESS1/LConn3 -- Three-Phase Breaker/LConn3
  a/RConn1 -- R_BESS1/RConn1
  R_BESS1/RConn2 -- b/RConn1
  c/RConn1 -- R_BESS1/RConn3

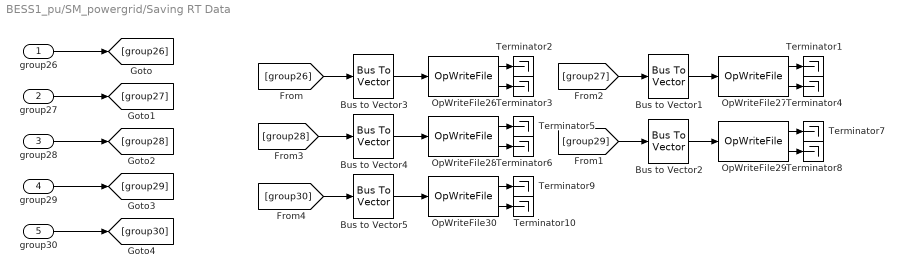
== system BESS1_pu/SM_powergrid/Saving RT Data ==
  group26 : Inport
  group27 : Inport  Port=2
  group28 : Inport  Port=3
  group29 : Inport  Port=4
  group30 : Inport  Port=5
  Bus to Vector{1..5} (5 alike) : BusToVector
  OpWriteFile26 : rtlab/DataLogging/OpWriteFile  Static_File=on  varname=BESS_m  Filename=BESS.mat  rtpath='./'  nrtpath='.\'  Acq_Group=26  file_size=(nls26+1)*8*(ld26/Ts)*1.5  write_offline=on  Sim_Mode=off  Nb_Samples=ld26/Ts  Buffer_size=(ld26/Ts)*8*(1+nls26)
      settings: SourceProductName=RT-LAB  Decimation=Decimation26
  OpWriteFile27 : rtlab/DataLogging/OpWriteFile  Static_File=on  varname=Grid_m  Filename=Grid.mat  rtpath='./'  nrtpath='.\'  Acq_Group=27  file_size=(nls27+1)*8*(ld27/Ts)*1.5  write_offline=on  Sim_Mode=off  Nb_Samples=ld27/Ts  Buffer_size=(ld26/Ts)*8*(1+nls26)
      settings: SourceProductName=RT-LAB  Decimation=Decimation27
  OpWriteFile28 : rtlab/DataLogging/OpWriteFile  Static_File=on  varname=cmd_isla  Filename=cmd_BRK.mat  rtpath='./'  nrtpath='.\'  Acq_Group=28  file_size=(nls28+1)*8*(ld28/Ts)*1.5  write_offline=on  Sim_Mode=off  Nb_Samples=ld28/Ts  Buffer_size=(ld28/Ts)*8*(1+nls28)
      settings: SourceProductName=RT-LAB  Decimation=Decimation28
  OpWriteFile29 : rtlab/DataLogging/OpWriteFile  Static_File=on  varname=Vabc_L  Filename=Vabc_L.mat  rtpath='./'  nrtpath='.\'  Acq_Group=29  file_size=(nls29+1)*8*(ld29/Ts)*1.5  write_offline=on  Sim_Mode=off  Nb_Samples=ld29/Ts  Buffer_size=(ld29/Ts)*8*(1+nls29)
      settings: SourceProductName=RT-LAB  Decimation=Decimation29
  OpWriteFile30 : rtlab/DataLogging/OpWriteFile  Static_File=on  varname=Iabc_L  Filename=Iabc_L.mat  rtpath='./'  nrtpath='.\'  Acq_Group=30  file_size=(nls30+1)*8*(ld30/Ts)*1.5  write_offline=on  Sim_Mode=off  Nb_Samples=ld30/Ts  Buffer_size=(ld30/Ts)*8*(1+nls30)
      settings: SourceProductName=RT-LAB  Decimation=Decimation30
  Terminator{1..10} (10 alike) : Terminator
  wires:
  OpWriteFile28/2 -> Terminator6/1
  OpWriteFile27/1 -> Terminator1/1
  OpWriteFile26/2 -> Terminator3/1
  OpWriteFile26/1 -> Terminator2/1
  OpWriteFile30/1 -> Terminator9/1
  OpWriteFile27/2 -> Terminator4/1
  OpWriteFile29/2 -> Terminator8/1
  OpWriteFile30/2 -> Terminator10/1
  OpWriteFile29/1 -> Terminator7/1
  OpWriteFile28/1 -> Terminator5/1
  group26/1 -> [group26]
  group27/1 -> [group27]
  group28/1 -> [group28]
  group29/1 -> [group29]
  group30/1 -> [group30]
  [group27] -> Bus to Vector1/1
  Bus to Vector1/1 -> OpWriteFile27/1
  [group29] -> Bus to Vector2/1
  Bus to Vector2/1 -> OpWriteFile29/1
  [group26] -> Bus to Vector3/1
  Bus to Vector3/1 -> OpWriteFile26/1
  [group28] -> Bus to Vector4/1
  Bus to Vector4/1 -> OpWriteFile28/1
  [group30] -> Bus to Vector5/1
  Bus to Vector5/1 -> OpWriteFile30/1

== system BESS1_pu/SM_powergrid/Subsystem1 ==
  V : Inport
  I : Inport  Port=2
  Gain : Gain  Gain=1/1e3
  Gain1 : Gain  Gain=1/1e3
  Power Measurement (Three-Phase) : eePowerMeasurement/Power Measurement (Three-Phase)  LabelModeActiveChoice=Continuous  F=60  K=[1]  Seq=Positive  Ts=0
      settings: SourceProductBaseCode=PS
  P(kW) : Outport
  Q(kW) : Outport  Port=2
  wires:
  I/1 -> Power Measurement (Three-Phase)/2
  Power Measurement (Three-Phase)/1 -> Gain/1
  Gain/1 -> P(kW)/1
  V/1 -> Power Measurement (Three-Phase)/1
  Power Measurement (Three-Phase)/2 -> Gain1/1
  Gain1/1 -> Q(kW)/1

== system BESS1_pu/SM_powergrid/BESS1/I_measurement ==
  Current Measurement : powerlib/Measurements/Current Measurement  PhasorSimulation=off  OutputType=Complex  PSBequivalent=0
  Current Measurement1 : powerlib/Measurements/Current Measurement  PhasorSimulation=off  OutputType=Complex  PSBequivalent=0
  Current Measurement2 : powerlib/Measurements/Current Measurement  PhasorSimulation=off  OutputType=Complex  PSBequivalent=0
  Mux : Mux  Inputs=3
  a : PMIOPort  Side=Left
  Va : PMIOPort  Port=2  Side=Right
  b : PMIOPort  Port=3  Side=Left
  Vb : PMIOPort  Port=4  Side=Right
  c : PMIOPort  Port=5  Side=Left
  Vc : PMIOPort  Port=6  Side=Right
  Iabc : Outport
  wires:
  Current Measurement2/1 -> Mux/3
  Current Measurement/1 -> Mux/1
  Mux/1 -> Iabc/1
  Current Measurement1/1 -> Mux/2
  connections:
  b/RConn1 -- Current Measurement1/LConn1
  Current Measurement/RConn1 -- Va/RConn1
  Current Measurement2/LConn1 -- c/RConn1
  Current Measurement/LConn1 -- a/RConn1
  Current Measurement1/RConn1 -- Vb/RConn1
  Current Measurement2/RConn1 -- Vc/RConn1

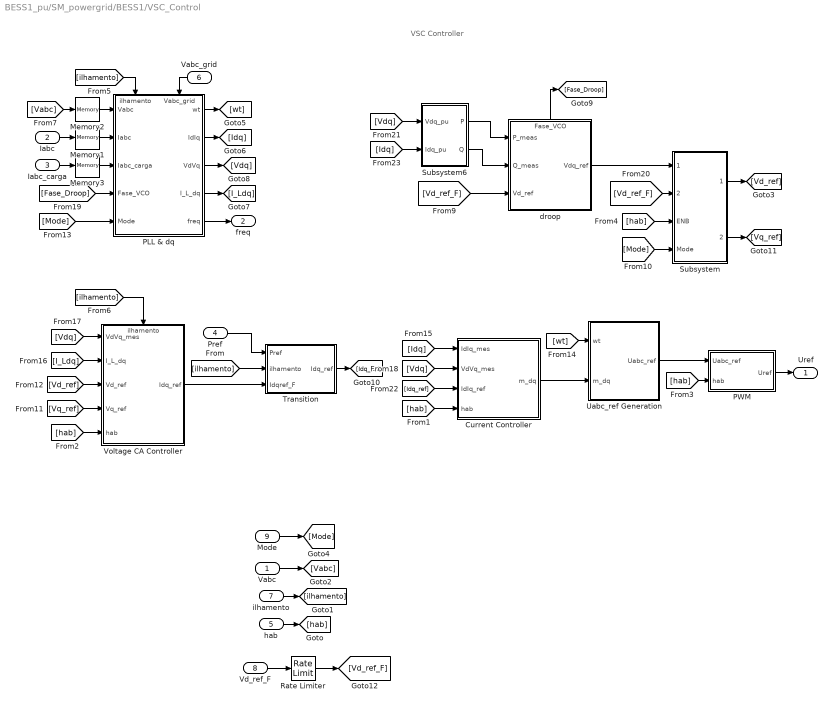
== system BESS1_pu/SM_powergrid/BESS1/VSC_Control ==
  note: VSC Controller
  Vabc : Inport  PortDimensions=3
  Iabc : Inport  Port=2  PortDimensions=3
  Iabc_carga : Inport  Port=3  PortDimensions=3
  Pref : Inport  Port=4
  hab : Inport  Port=5
  Vabc_grid : Inport  Port=6
  ilhamento : Inport  Port=7
  Vd_ref_F : Inport  Port=8
  Mode : Inport  Port=9
  Current Controller : Subsystem
  Memory1 : Memory
  Memory2 : Memory
  Memory3 : Memory
  PLL & dq : Subsystem
      settings: PortSchema="{\"entries\":[{\"content\":{\"sides\":[{\"content\":{\"connectorIds\":[\"In1\",\"In2\",\"In3\",\"In4\",\"In5\"]},\"type\":\"ConnectorPlacement.EquallySpacedRectSide\",\"uuid\":\"64d20dde-42ab-4edb-ad92-c6be12e892c7\"},{\"content\":{\"connectorIds\":[\"Out1\",\"Out2\",\"Out3\",\"Out4\",\"Out5\"],\"side\":\"RIGHT\"},\"type\":\"ConnectorPlacement.EquallySpacedRectSide\",\"uuid\":\"cd31aade-b06b-4739-a835-a1e701ab8abb\"},{\"content\":{\"connectorIds\":[\"In6\",\"In7\"],\"side\":\"TOP\"},\"type\":\"ConnectorPlacement.EquallySpacedRectSide\",\"uuid\":\"2701b331-cf72-43ae-9386-6ef3e97a40a4\"},{\"content\":{\"connectorIds\":[],\"side\":\"BOTTOM\"},\"type\":\"ConnectorPlacement.EquallySpacedRectSide\",\"uuid\":\"8be9bac3-2994-4daa-8fdc-f8992345cd0c\"},{\"content\":{\"connectorIds\":[],\"side\":\"HIDDEN\"},\"type\":\"ConnectorPlacement.EquallySpacedRectSide\",\"uuid\":\"1eae7d7b-5f10-4f62-8017-61451f815a0e\"}]},\"type\":\"ConnectorPlacement.EquallySpacedConnector\",\"uuid\":\"6d21a079-9214-47f9-9aac-c7feab4cf70a\"}],\"packageUris\":[\"http://schema.mathworks.com/mf0/Connector/R2020b\"],\"version\":\"1.0\"}"
  PWM : Subsystem
  Rate Limiter : RateLimiter  SampleTimeMode=inherited
  Subsystem : Subsystem
  Subsystem6 : Subsystem
  Transition : Subsystem
  "Uabc_ref Generation " : Subsystem
  Voltage CA Controller : Subsystem
      settings: PortSchema="{\"entries\":[{\"content\":{\"sides\":[{\"content\":{\"connectorIds\":[\"In1\",\"In2\",\"In3\",\"In4\",\"In5\"]},\"type\":\"ConnectorPlacement.EquallySpacedRectSide\",\"uuid\":\"c3c38183-e609-4bf9-bdc4-5d4c7430e475\"},{\"content\":{\"connectorIds\":[\"Out1\"],\"side\":\"RIGHT\"},\"type\":\"ConnectorPlacement.EquallySpacedRectSide\",\"uuid\":\"05b1c7df-f809-48a0-8491-c15ee0b7272f\"},{\"content\":{\"connectorIds\":[\"In6\"],\"side\":\"TOP\"},\"type\":\"ConnectorPlacement.EquallySpacedRectSide\",\"uuid\":\"846e9c8e-e4dc-4871-a4c5-784e7fc31652\"},{\"content\":{\"connectorIds\":[],\"side\":\"BOTTOM\"},\"type\":\"ConnectorPlacement.EquallySpacedRectSide\",\"uuid\":\"06fb89de-fa7d-4162-ac6c-729015011ca9\"},{\"content\":{\"connectorIds\":[],\"side\":\"HIDDEN\"},\"type\":\"ConnectorPlacement.EquallySpacedRectSide\",\"uuid\":\"45c6ff5f-148f-466a-b827-c6ac7d295801\"}]},\"type\":\"ConnectorPlacement.EquallySpacedConnector\",\"uuid\":\"a2520991-64a4-4b82-b28e-4f8bf2b520c6\"}],\"packageUris\":[\"http://schema.mathworks.com/mf0/Connector/R2020b\"],\"version\":\"1.0\"}"
  droop : Subsystem
      settings: PortSchema="{\"entries\":[{\"content\":{\"sides\":[{\"content\":{\"connectorIds\":[\"In1\",\"In2\",\"In3\"]},\"type\":\"ConnectorPlacement.EquallySpacedRectSide\",\"uuid\":\"c95e8b3e-35bd-48c8-8e50-04d46725ab46\"},{\"content\":{\"connectorIds\":[\"Out1\"],\"side\":\"RIGHT\"},\"type\":\"ConnectorPlacement.EquallySpacedRectSide\",\"uuid\":\"2e60c284-98da-4954-b6b2-cda2beb5c685\"},{\"content\":{\"connectorIds\":[\"Out2\"],\"side\":\"TOP\"},\"type\":\"ConnectorPlacement.EquallySpacedRectSide\",\"uuid\":\"c32118d3-fe15-4f6c-a8a8-a54172325389\"},{\"content\":{\"connectorIds\":[],\"side\":\"HIDDEN\"},\"type\":\"ConnectorPlacement.EquallySpacedRectSide\",\"uuid\":\"b212c9ba-9170-4332-93bb-c623da03332a\"}]},\"type\":\"ConnectorPlacement.EquallySpacedConnector\",\"uuid\":\"42409fcb-c65f-4db6-bf89-52ae480cc574\"}],\"packageUris\":[\"http://schema.mathworks.com/mf0/Connector/R2020b\"],\"version\":\"1.0\"}"
  Uref : Outport  VectorParamsAs1DForOutWhenUnconnected=off
  freq : Outport  Port=2
  wires:
  [Mode] -> PLL & dq/5(Mode)
  Mode/1 -> [Mode]
  [Vabc] -> Memory2/1
  Vabc/1 -> [Vabc]
  Subsystem6/2(Q) -> droop/2(Q_meas)
  Subsystem6/1(P) -> droop/1(P_meas)
  [Vd_ref_F] -> droop/3(Vd_ref)
  Vabc_grid/1 -> PLL & dq/7(Vabc_grid)
  [ilhamento] -> Voltage CA Controller/6(ilhamento)
  Voltage CA Controller/1(Idq_ref) -> Transition/3(Idqref_F)
  [ilhamento] -> Transition/2(ilhamento)
  Pref/1 -> Transition/1(Pref)
  PLL & dq/5(freq) -> freq/1
  [ilhamento] -> PLL & dq/6(ilhamento)
  ilhamento/1 -> [ilhamento]
  [hab] -> PWM/2(hab)
  Memory3/1 -> PLL & dq/3(Iabc_carga)
  Iabc_carga/1 -> Memory3/1
  [hab] -> Voltage CA Controller/5(hab)
  Memory2/1 -> PLL & dq/1(Vabc)
  Memory1/1 -> PLL & dq/2(Iabc)
  Iabc/1 -> Memory1/1
  hab/1 -> [hab]
  Current Controller/1(m_dq) -> "Uabc_ref Generation "/2(m_dq)
  "Uabc_ref Generation "/1(Uabc_ref) -> PWM/1(Uabc_ref)
  PWM/1(Uref) -> Uref/1
  [hab] -> Current Controller/4(hab)
  PLL & dq/1(wt) -> [wt]
  [wt] -> "Uabc_ref Generation "/1(wt)
  PLL & dq/2(IdIq) -> [Idq]
  [Idq] -> Current Controller/1(IdIq_mes)
  PLL & dq/4(I_L_dq) -> [I_Ldq]
  [I_Ldq] -> Voltage CA Controller/2(I_L_dq)
  PLL & dq/3(VdVq) -> [Vdq]
  [Vdq] -> Voltage CA Controller/1(VdVq_mes)
  [Vdq] -> Current Controller/2(VdVq_mes)
  droop/2("Fase_VCO ") -> [Fase_Droop]
  [Fase_Droop] -> PLL & dq/4("Fase_VCO ")
  [Vd_ref] -> Voltage CA Controller/3(Vd_ref)
  Transition/1(Idq_ref) -> [Idq_ref]
  [Idq_ref] -> Current Controller/3(IdIq_ref)
  droop/1("Vdq_ref ") -> Subsystem/1(Vdq_Droop)
  Subsystem/1(Vd_ref) -> [Vd_ref]
  [hab] -> Subsystem/3(ENB)
  [Mode] -> Subsystem/4(Mode)
  Subsystem/2(Vq_ref) -> [Vq_ref]
  [Vq_ref] -> Voltage CA Controller/4(Vq_ref)
  [Vd_ref_F] -> Subsystem/2(Vd_ref_F)
  [Vdq] -> Subsystem6/1(Vdq_pu)
  [Idq] -> Subsystem6/2(Idq_pu)
  Vd_ref_F/1 -> Rate Limiter/1
  Rate Limiter/1 -> [Vd_ref_F]

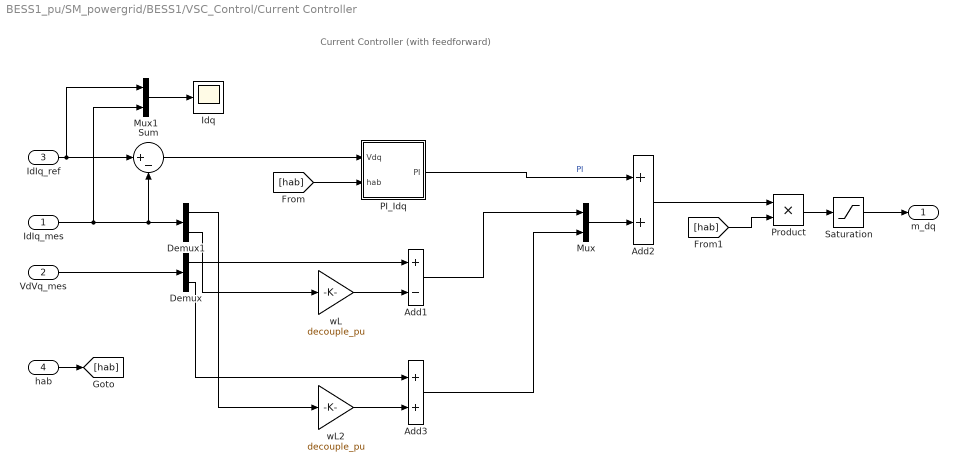
== system BESS1_pu/SM_powergrid/BESS1/VSC_Control/Current Controller ==
  note: Current Controller (with feedforward)
  IdIq_mes : Inport  PortDimensions=2
  VdVq_mes : Inport  Port=2  PortDimensions=2
  IdIq_ref : Inport  Port=3  PortDimensions=2
  hab : Inport  Port=4
  Add1 : Sum  Inputs=+-
  Add2 : Sum
  Add3 : Sum
  Demux : Demux  Outputs=2
  Demux1 : Demux  Outputs=2
  Idq : Scope
  Mux : Mux  Inputs=2
  Mux1 : Mux  Inputs=2
  PI_Idq : Subsystem
  Product : Product
  Saturation : Saturate  UpperLimit=10  LowerLimit=-10
  Sum : Sum  Inputs=|+-
  wL : Gain  Gain=decouple_pu  SaturateOnIntegerOverflow=on  OutDataTypeStr=Inherit: Same as input  ParamDataTypeStr=Inherit: Same as input
  wL2 : Gain  Gain=decouple_pu  SaturateOnIntegerOverflow=on  OutDataTypeStr=Inherit: Same as input  ParamDataTypeStr=Inherit: Same as input
  m_dq : Outport  VectorParamsAs1DForOutWhenUnconnected=off
  wires:
  Saturation/1 -> m_dq/1
  Product/1 -> Saturation/1
  IdIq_mes/1 -> Demux1/1, Sum/2, Mux1/2
  IdIq_ref/1 -> Sum/1, Mux1/1
  Mux1/1 -> Idq/1
  [hab] -> Product/2
  [hab] -> PI_Idq/2(hab)
  hab/1 -> [hab]
  Add2/1 -> Product/1
  Add3/1 -> Mux/2
  Demux/2 -> Add3/1
  Add1/1 -> Mux/1
  wL2/1 -> Add3/2
  Demux1/2 -> wL/1
  Demux1/1 -> wL2/1
  Demux/1 -> Add1/1
  VdVq_mes/1 -> Demux/1
  Sum/1 -> PI_Idq/1(Vdq)
  PI_Idq/1(PI) -> Add2/1  "PI"
  Mux/1 -> Add2/2
  wL/1 -> Add1/2

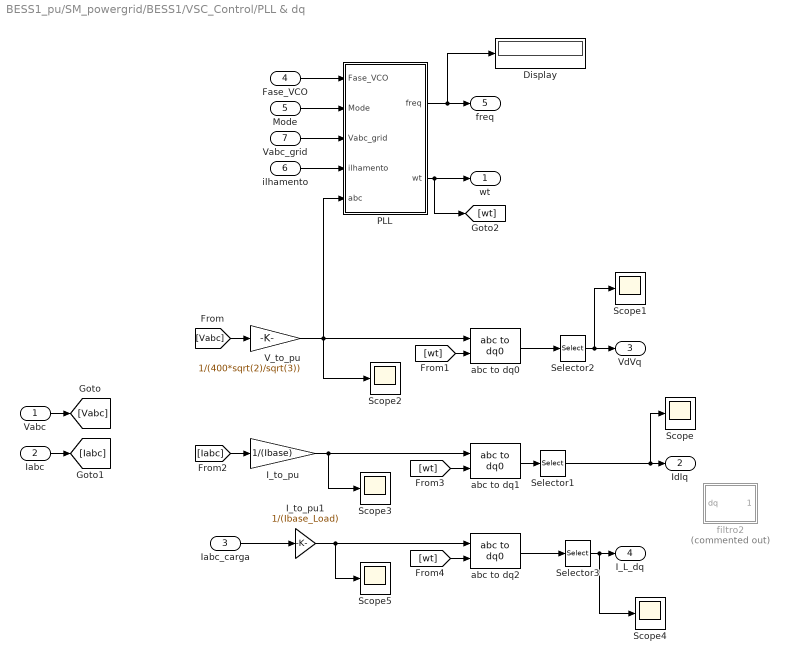
== system BESS1_pu/SM_powergrid/BESS1/VSC_Control/PLL & dq ==
  Vabc : Inport
  Iabc : Inport  Port=2
  Iabc_carga : Inport  Port=3
  "Fase_VCO " : Inport  Port=4
  Mode : Inport  Port=5
  ilhamento : Inport  Port=6
  Vabc_grid : Inport  Port=7
  Display : Display
  I_to_pu : Gain  Gain=1/(Ibase)  SaturateOnIntegerOverflow=on  OutDataTypeStr=Inherit: Same as input  ParamDataTypeStr=Inherit: Same as input
  I_to_pu1 : Gain  Gain=1/(Ibase_Load)  SaturateOnIntegerOverflow=on  OutDataTypeStr=Inherit: Same as input  ParamDataTypeStr=Inherit: Same as input
  PLL : Subsystem
  Scope{,1..5} (6 alike) : Scope
  Selector1 : Selector  InputPortWidth=3  IndexOptions=Index vector (dialog)  Indices=[1 2]  OutputSizes=1
  Selector2 : Selector  InputPortWidth=3  IndexOptions=Index vector (dialog)  Indices=[1 2]  OutputSizes=1
  Selector3 : Selector  InputPortWidth=3  IndexOptions=Index vector (dialog)  Indices=[1 2]  OutputSizes=1
  V_to_pu : Gain  Gain=1/(400*sqrt(2)/sqrt(3))  SaturateOnIntegerOverflow=on  OutDataTypeStr=Inherit: Same as input  ParamDataTypeStr=Inherit: Same as input
  abc to dq0 : powerlib_meascontrol/Transformations/abc to dq0  Alignment=90 degrees behind phase A axis
  abc to dq1 : powerlib_meascontrol/Transformations/abc to dq0  Alignment=90 degrees behind phase A axis
  abc to dq2 : powerlib_meascontrol/Transformations/abc to dq0  Alignment=90 degrees behind phase A axis
  filtro2 : Subsystem  Commented=on
  wt : Outport  VectorParamsAs1DForOutWhenUnconnected=off
  IdIq : Outport  Port=2  VectorParamsAs1DForOutWhenUnconnected=off
  VdVq : Outport  Port=3  VectorParamsAs1DForOutWhenUnconnected=off
  I_L_dq : Outport  Port=4
  freq : Outport  Port=5  VectorParamsAs1DForOutWhenUnconnected=off
  wires:
  "Fase_VCO "/1 -> PLL/1("Fase_VCO ")
  [Iabc] -> I_to_pu/1
  Iabc/1 -> [Iabc]
  Vabc/1 -> [Vabc]
  Vabc_grid/1 -> PLL/3(Vabc_grid)
  PLL/1(freq) -> Display/1, freq/1
  PLL/2(wt) -> [wt], wt/1
  ilhamento/1 -> PLL/4(ilhamento)
  Selector3/1 -> Scope4/1, I_L_dq/1
  abc to dq2/1 -> Selector3/1
  Iabc_carga/1 -> I_to_pu1/1
  Selector2/1 -> VdVq/1, Scope1/1
  abc to dq0/1 -> Selector2/1
  abc to dq1/1 -> Selector1/1
  [Vabc] -> V_to_pu/1
  V_to_pu/1 -> Scope2/1, abc to dq0/1, PLL/5(abc)
  I_to_pu/1 -> Scope3/1, abc to dq1/1
  I_to_pu1/1 -> Scope5/1, abc to dq2/1
  Selector1/1 -> IdIq/1, Scope/1
  Mode/1 -> PLL/2(Mode)
  [wt] -> abc to dq0/2
  [wt] -> abc to dq1/2
  [wt] -> abc to dq2/2

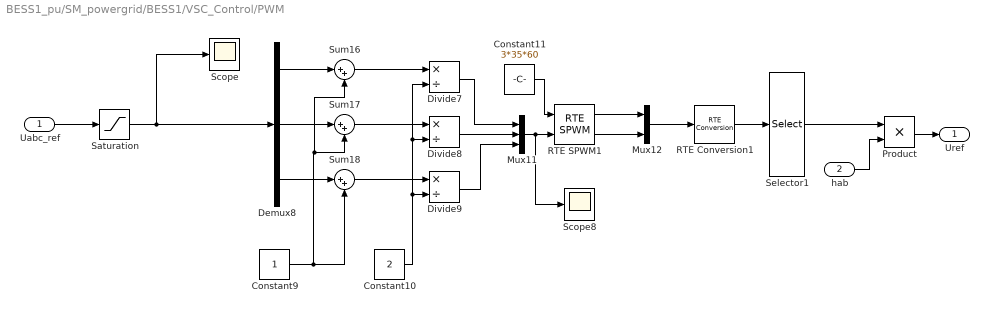
== system BESS1_pu/SM_powergrid/BESS1/VSC_Control/PWM ==
  Uabc_ref : Inport
  hab : Inport  Port=2
  Constant10 : Constant  Value=2
  Constant11 : Constant  Value=3*35*60
  Constant9 : Constant
  Demux8 : Demux  Outputs=3
  Divide7 : Product  Inputs=*/
  Divide8 : Product  Inputs=*/
  Divide9 : Product  Inputs=*/
  Mux11 : Mux  Inputs=3
  Mux12 : Mux  Inputs=2
  Product : Product
  RTE Conversion1 : rteventslib/Signal Attributes/RTE Conversion  inputdatatype=RTE Boolean  outputdatatype=Double  compensation=Enabled  nbMaxEvents=4  sampleTime=Ts
  RTE SPWM1 : rteventslib/Sources/RTE SPWM  NumberPhases=3-ph  CenterAlignmentMode=On  MaxFreq=inf  MinFreq=0  EnablingPort=off  ComplementaryMode=on  SpaceVector=off  RiseTimeDelay=0  MaxEvents=4  SampleTime=Ts
  Saturation : Saturate  UpperLimit=2  LowerLimit=-2
  Scope : Scope
  Scope8 : Scope
  Selector1 : Selector  InputPortWidth=6  IndexOptions=Index vector (dialog)  Indices=[1 4 2 5 3 6]  OutputSizes=1
  Sum16 : Sum  Inputs=|++
  Sum17 : Sum  Inputs=|++
  Sum18 : Sum  Inputs=|++
  Uref : Outport  VectorParamsAs1DForOutWhenUnconnected=off
  wires:
  hab/1 -> Product/2
  Product/1 -> Uref/1
  Selector1/1 -> Product/1
  Saturation/1 -> Demux8/1, Scope/1
  RTE SPWM1/1 -> Mux12/1
  Constant9/1 -> Sum18/2, Sum17/2, Sum16/2
  Constant11/1 -> RTE SPWM1/1
  Sum16/1 -> Divide7/1
  Constant10/1 -> Divide9/2, Divide8/2, Divide7/2
  Sum17/1 -> Divide8/1
  Divide9/1 -> Mux11/3
  RTE SPWM1/2 -> Mux12/2
  Uabc_ref/1 -> Saturation/1
  Demux8/2 -> Sum17/1
  Divide8/1 -> Mux11/2
  Sum18/1 -> Divide9/1
  Mux11/1 -> RTE SPWM1/2, Scope8/1
  Divide7/1 -> Mux11/1
  Demux8/1 -> Sum16/1
  Demux8/3 -> Sum18/1
  Mux12/1 -> RTE Conversion1/1
  RTE Conversion1/1 -> Selector1/1

== system BESS1_pu/SM_powergrid/BESS1/VSC_Control/Subsystem ==
  Vdq_Droop : Inport
  Vd_ref_F : Inport  Port=2
  ENB : Inport  Port=3
  Mode : Inport  Port=4
  Constant : Constant  Value=0
  Demux : Demux  Outputs=2
  Product : Product
  Switch : Switch  Criteria=u2 > Threshold  Threshold=1.5
  Switch1 : Switch  Criteria=u2 > Threshold  Threshold=1.5
  Vd_ref : Outport
  Vq_ref : Outport  Port=2
  wires:
  [Mode] -> Switch/2
  [Mode] -> Switch1/2
  [Vd_ref] -> Switch/1
  Switch1/1 -> Vq_ref/1
  Constant/1 -> Switch1/1
  [Vq_ref_Droop] -> Switch1/3
  Vd_ref_F/1 -> Product/1
  Product/1 -> [Vd_ref]
  [hab] -> Product/2
  ENB/1 -> [hab]
  Switch/1 -> Vd_ref/1
  Vdq_Droop/1 -> Demux/1
  Demux/1 -> [Vd_ref_Droop]
  Demux/2 -> [Vq_ref_Droop]
  [Vd_ref_Droop] -> Switch/3
  Mode/1 -> [Mode]
